simulink library "pmm"  (R2021b)
settings: Solver=VariableStepAuto  StartTime=0.0  StopTime=10.0  RelTol=1e-3
undefined symbols (not defined in the file or in its folder): APMM_CoolgFanActCurr_X_pct, APMM_EWP1Curr_X_c, APMM_EWP3Curr_X_c, APMM_LVBattChktime_X_enum, APMM_LVBattChrgtime_X_enum, APMM_LVChrgLv24V_X_mV, APMM_LVChrgLv_X_mV, ENUM_ANTITHEFT_ALARM, ENUM_ANTITHEFT_ARM, ENUM_ANTITHEFT_DISARM, ENUM_ANTITHEFT_WAIT, ENUM_CHRGPLUGSTA_NONE, ENUM_CRASHSTATE_NOCRASH, ENUM_DCDCFAULTSTA_ANYFAULTLV1, ENUM_DCDCFAULTSTA_ANYFAULTLV2, ENUM_DRIVETRAIN_AWD, ENUM_DRIVETRAIN_FWD, ENUM_DRIVETRAIN_RWD, ENUM_EBSBRKSW_PRESSED, ENUM_GEARACTUALPOSN_D, ENUM_GEARACTUALPOSN_N, ENUM_GEARACTUALPOSN_P, ENUM_GEARACTUALPOSN_R, ENUM_HVBATTREADYPRE_READY, ENUM_PDKEYRAWLULOCK_INLOCK, ENUM_PDKEYRAWLULOCK_INUNLOCK, ENUM_PDKEYRAWPS_INPS, ENUM_PDKEYSTA_LOCK, ENUM_PDKEYSTA_PS, ENUM_PDKEYSTA_UNAVALIABLE, ENUM_PDKEYSTA_UNLOCK, ENUM_POWERSTA_OFF, ENUM_POWERSTA_OFFA, ENUM_POWERSTA_OFFC, ENUM_POWERSTA_ON, ENUM_POWERSTA_READY, ENUM_POWERSTA_STANDBY, ENUM_PWRSTASW_PWRUP, ENUM_PWRSTASW_READY, FALSE, KPMM_AllDoorClosedHoldTime_s, KPMM_APSAllowThd_pct, KPMM_BattDownFailtime_s, KPMM_BattUpFailtime_s, KPMM_BattUpResetRty_cnt, KPMM_BattUpResetSW_flg, KPMM_BattUpResetTO_s, KPMM_BattUpRstDlyTO_s, KPMM_BrakeSWHoldTime_s, KPMM_ChrgPlugHoldTime_s, KPMM_DCDCDisableFailtime_s, KPMM_DCDCEnableFailtime_s, KPMM_DCDCVSET_V, KPMM_DCDCVSETLVChrg_V, KPMM_DoorSWHoldTime_s, KPMM_DriverSafetyChkFailtime_s, KPMM_DrivetrainSelect_enum_ovrdflg, KPMM_DrivetrainSelect_enum_ovrdval, KPMM_FDADC12VDetAccu_s, KPMM_FDADC12VDetAccuIntval_s ... (+60)
libraries: simulink x35, hcu_lib x13
(part 4 of 6)

== stateflow chart pmm/PMM/PMM/RequirementManagementForPowerStateConstrain ==
  state RequirementManagementForPowerStateConstrain
    (default) -> (junction 2) : {VPMM_TCountSta_enum = ENUM_TCOUNTSTA_NOCOUNTING;
        |  VPMM_PwrOffTimer_s = 0;}
    RequirementManagementForPowerStateConstrain -> (junction 2) [order 2]
    (junction 2) -> (junction 3) : {VPMM_PwrStaConstraint_enum = ENUM_PWRCONSTRAINT_NOREQUEST;}
    RequirementManagementForPowerStateConstrain -> (junction 3) [order 1] : [VPMM_ConstraintLoop_flg]
        | {VPMM_ConstraintLoop_flg = FALSE;}
    (junction 3) -> (junction 4) [order 1] : [VPMM_PowerSta_enum == ENUM_POWERSTA_ON || ...
        |  VPMM_PowerSta_enum == ENUM_POWERSTA_OFFA || ...
        |  VPMM_PowerSta_enum == ENUM_POWERSTA_OFFC]
    (junction 4) -> (junction 5) [order 1] : [VINP_PwrReq_OTA_enum == ENUM_PWRREQOTA_REQPOWERON || ...
        |  VINP_OFFACMODE_enum == ENUM_OFFACMODE_CAMP]
    (junction 3) -> (junction 6) [order 2]
    (junction 4) -> (junction 7) [order 2]
    (junction 5) -> (junction 8) : {VPMM_PwrStaConstraint_enum = ENUM_PWRCONSTRAINT_PWRSTAON;}
    (junction 7) -> (junction 8) [order 1] : [VINP_AVMOFFRecButt_flg == ENUM_AVMOFFRECBUTT_ON || ...
        |  VINP_OFFACMODE_enum == ENUM_OFFACMODE_PET || ...
        |  VINP_OFFACMODE_enum == ENUM_OFFACMODE_ON || ...
        |  VINP_HVBPreheatPrecoolSta_enum == ENUM_HVBPRESTA_PREHEAT || ...
        |  VINP_HVBPreheatPrecoolSta_enum == ENUM_HVBPRESTA_PRECOOL]
        | {VPMM_PwrStaConstraint_enum = ENUM_PWRCONSTRAINT_HVACTIVE;}
    (junction 7) -> (junction 80) [order 2]
    (junction 8) -> (junction 9) : {VPMM_TCountSta_enum = ENUM_TCOUNTSTA_NOCOUNTING;
        |  VPMM_PwrOffTimer_s = 0;
        |  VPMM_ConstraintLoop_flg = TRUE;}
    (junction 80) -> (junction 82) [order 1] : [VPMM_TCountSta_enum == ENUM_TCOUNTSTA_COUNTINGFINISH]
    (junction 82) -> (junction 90) [order 1] : [VPMM_PwrStaSW_enum == ENUM_PWRSTASW_PWRDOWN]
    (junction 80) -> (junction 10) [order 2]
    (junction 82) -> (junction 84) [order 2]
    (junction 90) -> (junction 92) : {VPMM_TCountSta_enum = ENUM_TCOUNTSTA_NOCOUNTING;}
    (junction 10) -> (junction 11) [order 1] : [(VPMM_PowerOffTSet_s > 0 && ...
        |   (VINP_RePwrReqTbox_enum == ENUM_REPWRREQTBOX_REQVEHCHK || ...
        |    VINP_RePwrReqTbox_enum == ENUM_REPWRREQTBOX_REQDTC || ...
        |    VINP_RePwrReqTbox_enum == ENUM_REPWRREQTBOX_REQRADIO || ...
        |    VINP_RePwrReqTbox_enum == ENUM_REPWRREQTBOX_REQON)) || ...
        |  (VPMM_PowerOffTSetDKC_enum > 0 && ...
        |   (VINP_RePwrReqDKCT_enum == ENUM_REPWRREQDKC_REQVEHCHK || ...
        |    VINP_RePwrReqDKCT_enum == ENUM_REPWRREQDKC_REQDTC || ...
        |    VINP_RePwrReqDKCT_enum == ENUM_REPWRREQDKC_REQRADIO || ...
        |    VINP_RePwrReqDKCT_enum == ENUM_REPWRREQDKC_REQON))]
    (junction 10) -> (junction 12) [order 2]
    (junction 11) -> (junction 13) : {VPMM_PwrStaConstraint_enum = ENUM_PWRCONSTRAINT_ONFORTIME;}
    (junction 12) -> (junction 13) [order 1] : [(VPMM_PowerOffTSet_s > 0 && ...
        |   VINP_RePwrReqTbox_enum == ENUM_REPWRREQTBOX_REQACTEMP) || ...
        |  (VPMM_PowerOffTSetDKC_enum > 0 && ...
        |   VINP_RePwrReqDKCT_enum == ENUM_REPWRREQDKC_REQACTEMP)]
        | {VPMM_PwrStaConstraint_enum = ENUM_PWRCONSTRAINT_HVFORTIME;}
    (junction 13) -> (junction 14) [order 1] : [(VPMM_PowerOffTSet_s >= VPMM_PowerOffTSetDKC_enum && VPMM_PwrOffTimer_s >= VPMM_PowerOffTSet_s) || ...
        |  (VPMM_PowerOffTSetDKC_enum > VPMM_PowerOffTSet_s && VPMM_PwrOffTimer_s >= VPMM_PowerOffTSetDKC_enum)]
    (junction 12) -> (junction 15) [order 2] : {VPMM_TCountSta_enum = ENUM_TCOUNTSTA_NOCOUNTING;
        |  VPMM_PwrOffTimer_s = 0;}
    (junction 13) -> (junction 16) [order 2] : {VPMM_TCountSta_enum = ENUM_TCOUNTSTA_TIMMERCOUNTING;
        |  VPMM_PwrOffTimer_s += task_time_s;
        |  VPMM_ConstraintLoop_flg = TRUE;}
    (junction 14) -> (junction 17) : {VPMM_TCountSta_enum = ENUM_TCOUNTSTA_COUNTINGFINISH;
        |  VPMM_PwrStaConstraint_enum = ENUM_PWRCONSTRAINT_NOREQUEST;
        |  VPMM_PwrOffTimer_s = 0;}
  data: task_time_s input; VPMM_PowerSta_enum input; VINP_AVMOFFRecButt_flg input; VINP_HVBPreheatPrecoolSta_enum input; VINP_OFFACMODE_enum input; VPMM_PowerOffTSet_s input; VPMM_PowerOffTSetDKC_enum input; VINP_PwrReq_OTA_enum input; VINP_RePwrReqDKCT_enum input; VINP_RePwrReqTbox_enum input; VPMM_PwrStaConstraint_enum output; VPMM_TCountSta_enum output; VPMM_PwrOffTimer_s local single; ENUM_AVMOFFRECBUTT_ON parameter; ENUM_HVBPRESTA_PRECOOL parameter; ENUM_HVBPRESTA_PREHEAT parameter; ENUM_OFFACMODE_CAMP parameter; ENUM_OFFACMODE_ON parameter; ENUM_OFFACMODE_PET parameter; ENUM_POWERSTA_OFFA parameter; ENUM_POWERSTA_OFFC parameter; ENUM_POWERSTA_ON parameter; ENUM_PWRCONSTRAINT_HVACTIVE parameter; ENUM_PWRCONSTRAINT_HVFORTIME parameter; ENUM_PWRCONSTRAINT_NOREQUEST parameter; ENUM_PWRCONSTRAINT_ONFORTIME parameter; ENUM_PWRCONSTRAINT_PWRSTAON parameter; ENUM_PWRREQOTA_REQPOWERON parameter; ENUM_REPWRREQDKC_REQACTEMP parameter; ENUM_REPWRREQDKC_REQDTC parameter; ENUM_REPWRREQDKC_REQON parameter; ENUM_REPWRREQDKC_REQRADIO parameter; ENUM_REPWRREQDKC_REQVEHCHK parameter; ENUM_REPWRREQTBOX_REQACTEMP parameter; ENUM_REPWRREQTBOX_REQDTC parameter; ENUM_REPWRREQTBOX_REQON parameter; ENUM_REPWRREQTBOX_REQRADIO parameter; ENUM_REPWRREQTBOX_REQVEHCHK parameter; ENUM_TCOUNTSTA_COUNTINGFINISH parameter; ENUM_TCOUNTSTA_NOCOUNTING parameter; ENUM_TCOUNTSTA_TIMMERCOUNTING parameter; VPMM_ConstraintLoop_flg local boolean; FALSE parameter; TRUE parameter; VPMM_PwrStaSW_enum input; ENUM_PWRSTASW_PWRDOWN parameter
